simulink model "Xi_D_D_C"  (R2018b)
settings: Solver=VariableStepAuto  StartTime=0.0  StopTime=10.0  RelTol=1e-3
settings Model: Creator=lingchenyang  LastModifiedBy=lingchenyang

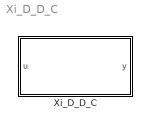
== system Xi_D_D_C ==
  "Xi_D_D_C " : MATLAB Function  TreatAsAtomicUnit=on

== matlab function Xi_D_D_C/Xi_D_D_C  ==
  data: u input; y output
function y = fcn(u)

y = [0,-u(3), u(2),0,0,0;
    u(3),0,-u(1),0,0,0;
    -u(2),u(1),0,0,0,0;
    0,0,0,-u(2),0,0;
    0,0,0,0,0,0;
    0,0,0,0,0,0;
    0,0,0,0,0,0;
    0,0,0,-u(3),0,0;
    0,0,0,0,0,0;
    0,0,0,0,0,0;
    0,0,0,u(1),0,0;
    0,0,0,0,0,0;
    0,0,0,0,0,0;
    0,0,0,0,0,0;
    0,0,0,u(2),0,0;
    0,0,0,0,u(3),0;
    0,0,0,0,0,0;
    0,0,0,0,0,0;
    0,0,0,0,-u(1),0;
    0,0,0,0,0,0;
    0,0,0,0,0,0;
    0,0,0,0,0,0;
    0,0,0,0,0,0;
    0,0,0,0,u(3),0;
    0,0,0,0,0,0;
    0,0,0,0,0,0;
    0,0,0,0,-u(1),0;
    0,0,0,0,0,-u(2);
    0,0,0,0,0,0;
    0,0,0,0,0,0;
    0,0,0,0,0,0;
    0,0,0,0,0,-u(3);
    0,0,0,0,0,0;
    0,0,0,0,0,0;
    0,0,0,0,0,u(1);
    0,0,0,0,0,0;
    0,0,0,0,0,0;
    0,0,0,0,0,0;
    0,0,0,0,0,u(2)];
